simulink model "tracked_vehicle"  (R2026a)
settings: configuration reference "standardSILConfiguraitonParams" (kept outside this file)
undefined symbols (not defined in the file): vehicleParams
settings Model: Creator=jerem  LastModifiedBy=Edison Altamirano
settings ConfigSetRef: SourceName=standardSILConfiguraitonParams  SourceLocation=Base Workspace

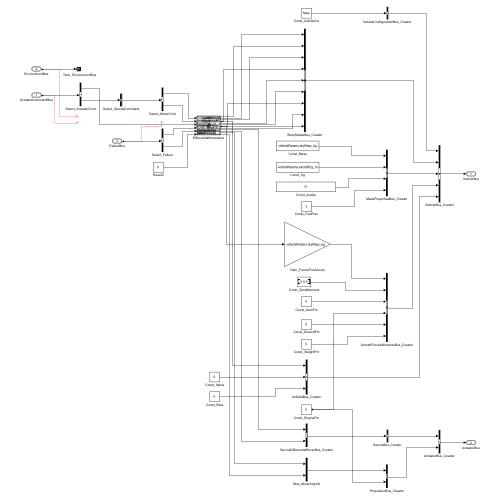
[thumbnail: Simulink's stored preview of the top-level diagram]
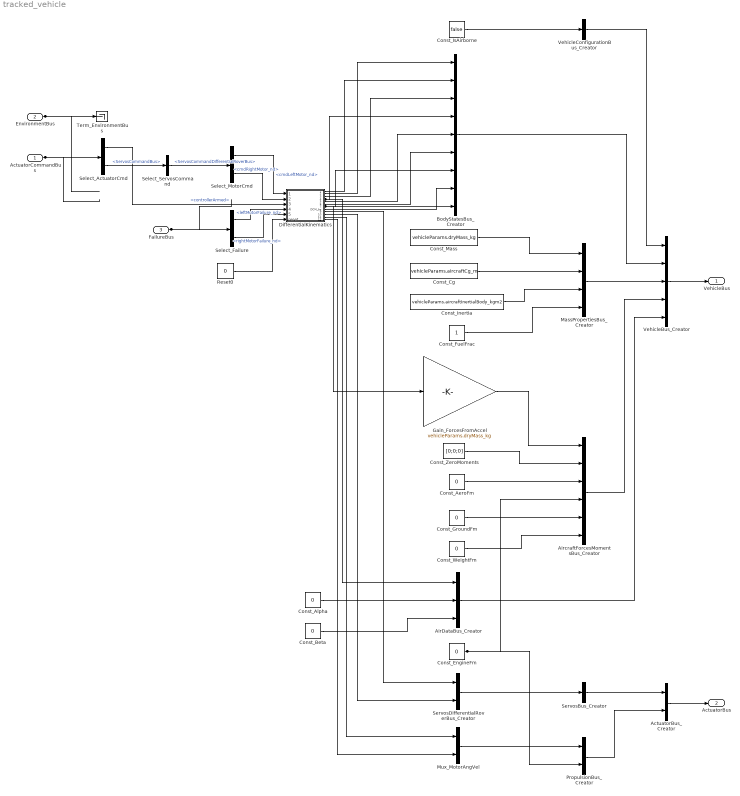
== system tracked_vehicle ==
  ActuatorCommandBus : Inport  OutDataTypeStr=Bus: ActuatorCommandBus
  EnvironmentBus : Inport  Port=2  OutDataTypeStr=Bus: EnvironmentBus
  FailureBus : Inport  Port=3  OutDataTypeStr=Bus: FailureBus
  ActuatorBus_Creator : BusCreator  Inputs=2  OutDataTypeStr=Bus: ActuatorBus
  AirDataBus_Creator : BusCreator  Inputs=3  OutDataTypeStr=Bus: AirDataBus
  AircraftForcesMomentsBus_Creator : BusCreator  Inputs=6  OutDataTypeStr=Bus: AircraftForcesMomentsBus
  BodyStatesBus_Creator : BusCreator  Inputs=9  OutDataTypeStr=Bus: BodyStateBus
  Const_AeroFm : Constant  Value=0  OutDataTypeStr=Bus: ComponentForcesMomentsBus
  Const_Alpha : Constant  Value=0
  Const_Beta : Constant  Value=0
  Const_Cg : Constant  Value=vehicleParams.aircraftCg_m
  Const_EngineFm : Constant  Value=0  OutDataTypeStr=Bus: ComponentForcesMomentsBus
  Const_FuelFrac : Constant
  Const_GroundFm : Constant  Value=0  OutDataTypeStr=Bus: ComponentForcesMomentsBus
  Const_Inertia : Constant  Value=vehicleParams.aircraftInertialBody_kgm2
  Const_IsAirborne : Constant  Value=false  OutDataTypeStr=boolean
  Const_Mass : Constant  Value=vehicleParams.dryMass_kg
  Const_WeightFm : Constant  Value=0  OutDataTypeStr=Bus: ComponentForcesMomentsBus
  Const_ZeroMoments : Constant  Value=[0;0;0]
  DifferentialKinematics : MATLAB Function  TreatAsAtomicUnit=on
  Gain_ForcesFromAccel : Gain  Gain=vehicleParams.dryMass_kg
  MassPropertiesBus_Creator : BusCreator  Inputs=4  OutDataTypeStr=Bus: MassPropertiesBus
  Mux_MotorAngVel : Mux  Inputs=2
  PropulsionBus_Creator : BusCreator  Inputs=2  OutDataTypeStr=Bus: PropulsionBus
  Reset0 : Constant  Value=0
  Select_ActuatorCmd : BusSelector  OutputSignals=controllerArmed,ServosCommandBus
  Select_Failure : BusSelector  OutputSignals=leftMotorFailure_nd,rightMotorFailure_nd
  Select_MotorCmd : BusSelector  OutputSignals=cmdLeftMotor_nd,cmdRightMotor_nd
  Select_ServosCommand : BusSelector  OutputSignals=ServosCommandDifferentialRoverBus
  ServosBus_Creator : BusCreator  Inputs=1  OutDataTypeStr=Bus: ServosBus
  ServosDifferentialRoverBus_Creator : BusCreator  Inputs=2  OutDataTypeStr=Bus: ServosDifferentialRoverBus
  Term_EnvironmentBus : Terminator
  VehicleBus_Creator : BusCreator  Inputs=5  OutDataTypeStr=Bus: VehicleBus
  VehicleConfigurationBus_Creator : BusCreator  Inputs=1  OutDataTypeStr=Bus: VehicleConfigurationBus
  VehicleBus : Outport  OutDataTypeStr=Bus: VehicleBus
  ActuatorBus : Outport  Port=2  OutDataTypeStr=Bus: ActuatorBus
  wires:
  EnvironmentBus/1 -> Term_EnvironmentBus/1
  ActuatorCommandBus/1 -> Select_ActuatorCmd/1
  Const_Mass/1 -> MassPropertiesBus_Creator/1
  Select_ServosCommand/1 -> Select_MotorCmd/1  "<ServosCommandDifferentialRoverBus>"
  Select_ActuatorCmd/1 -> DifferentialKinematics/3(controllerArmed)  "<controllerArmed>"
  Select_ActuatorCmd/2 -> Select_ServosCommand/1  "<ServosCommandBus>"
  Const_Inertia/1 -> MassPropertiesBus_Creator/3
  FailureBus/1 -> Select_Failure/1
  Select_MotorCmd/2 -> DifferentialKinematics/2(cmdRightMotor_nd)  "<cmdRightMotor_nd>"
  PropulsionBus_Creator/1 -> ActuatorBus_Creator/2
  Select_MotorCmd/1 -> DifferentialKinematics/1(cmdLeftMotor_nd)  "<cmdLeftMotor_nd>"
  Select_Failure/1 -> DifferentialKinematics/4(leftMotorFailure_nd)  "<leftMotorFailure_nd>"
  DifferentialKinematics/10(rightWheelSpeed_radps) -> ServosDifferentialRoverBus_Creator/2
  Select_Failure/2 -> DifferentialKinematics/5(rightMotorFailure_nd)  "<rightMotorFailure_nd>"
  Reset0/1 -> DifferentialKinematics/6(reset)
  DifferentialKinematics/1(posNED_m) -> BodyStatesBus_Creator/2
  DifferentialKinematics/2(velNED_mps) -> BodyStatesBus_Creator/1
  DifferentialKinematics/3(eulerAngles_rad) -> BodyStatesBus_Creator/3
  DifferentialKinematics/4(velBody_mps) -> BodyStatesBus_Creator/4, AirDataBus_Creator/1
  AircraftForcesMomentsBus_Creator/1 -> VehicleBus_Creator/4
  Const_EngineFm/1 -> AircraftForcesMomentsBus_Creator/4, PropulsionBus_Creator/2
  DifferentialKinematics/5(angVelBody_radps) -> BodyStatesBus_Creator/5
  DifferentialKinematics/9(leftWheelSpeed_radps) -> ServosDifferentialRoverBus_Creator/1
  DifferentialKinematics/6(angAccelBody_radps2) -> BodyStatesBus_Creator/6
  DifferentialKinematics/7(accelBody_mps2) -> BodyStatesBus_Creator/9, BodyStatesBus_Creator/7, Gain_ForcesFromAccel/1
  DifferentialKinematics/8(DCM_be) -> BodyStatesBus_Creator/8
  VehicleConfigurationBus_Creator/1 -> VehicleBus_Creator/1
  DifferentialKinematics/11(leftMotorAngVel_radps) -> Mux_MotorAngVel/1
  DifferentialKinematics/12(rightMotorAngVel_radps) -> Mux_MotorAngVel/2
  Const_WeightFm/1 -> AircraftForcesMomentsBus_Creator/6
  Const_Alpha/1 -> AirDataBus_Creator/2
  Const_Beta/1 -> AirDataBus_Creator/3
  Const_IsAirborne/1 -> VehicleConfigurationBus_Creator/1
  BodyStatesBus_Creator/1 -> VehicleBus_Creator/2
  Const_Cg/1 -> MassPropertiesBus_Creator/2
  Const_GroundFm/1 -> AircraftForcesMomentsBus_Creator/5
  Const_FuelFrac/1 -> MassPropertiesBus_Creator/4
  ServosBus_Creator/1 -> ActuatorBus_Creator/1
  Gain_ForcesFromAccel/1 -> AircraftForcesMomentsBus_Creator/1
  Const_ZeroMoments/1 -> AircraftForcesMomentsBus_Creator/2
  Const_AeroFm/1 -> AircraftForcesMomentsBus_Creator/3
  AirDataBus_Creator/1 -> VehicleBus_Creator/5
  ServosDifferentialRoverBus_Creator/1 -> ServosBus_Creator/1
  Mux_MotorAngVel/1 -> PropulsionBus_Creator/1
  VehicleBus_Creator/1 -> VehicleBus/1
  MassPropertiesBus_Creator/1 -> VehicleBus_Creator/3
  ActuatorBus_Creator/1 -> ActuatorBus/1

== matlab function tracked_vehicle/DifferentialKinematics ==
  data: cmdLeftMotor_nd input; posNED_m output; cmdRightMotor_nd input; controllerArmed input; leftMotorFailure_nd input; rightMotorFailure_nd input; reset input; velNED_mps output; eulerAngles_rad output; velBody_mps output; angVelBody_radps output; angAccelBody_radps2 output; accelBody_mps2 output; DCM_be output; leftWheelSpeed_radps output; rightWheelSpeed_radps output; leftMotorAngVel_radps output; rightMotorAngVel_radps output
function [posNED_m, velNED_mps, eulerAngles_rad, velBody_mps, angVelBody_radps, angAccelBody_radps2, accelBody_mps2, DCM_be, leftWheelSpeed_radps, rightWheelSpeed_radps, leftMotorAngVel_radps, rightMotorAngVel_radps] = DifferentialKinematics(cmdLeftMotor_nd, cmdRightMotor_nd, controllerArmed, leftMotorFailure_nd, rightMotorFailure_nd, reset)
%#codegen
persistent posN posE yaw leftSpeed rightSpeed
if isempty(posN) || reset
    posN = 0; posE = 0; yaw = 1.9199; leftSpeed = 0; rightSpeed = 0;
end
Ts = 0.004;
trackWidth_m = 1.5;
wheelRadius_m = 0.3;
maxSpeed_mps = 3.0;
tauMotor_s = 0.6;
referenceAltitude_m = 116 * 0.3048;
if leftMotorFailure_nd || ~controllerArmed
    leftCmd_mps = 0;
else
    leftCmd_mps = cmdLeftMotor_nd * maxSpeed_mps;
end
if rightMotorFailure_nd || ~controllerArmed
    rightCmd_mps = 0;
else
    rightCmd_mps = cmdRightMotor_nd * maxSpeed_mps;
end
leftDot = (leftCmd_mps - leftSpeed) / tauMotor_s;
rightDot = (rightCmd_mps - rightSpeed) / tauMotor_s;
v = (leftSpeed + rightSpeed) / 2;
yawRate = (rightSpeed - leftSpeed) / trackWidth_m;
posN = posN + Ts * v * cos(yaw);
posE = posE + Ts * v * sin(yaw);
yaw = yaw + Ts * yawRate;
leftSpeed = leftSpeed + Ts * leftDot;
rightSpeed = rightSpeed + Ts * rightDot;
posNED_m = [posN; posE; -referenceAltitude_m];
velNED_mps = [v*cos(yaw); v*sin(yaw); 0];
eulerAngles_rad = [0; 0; yaw];
velBody_mps = [v; 0; 0];
angVelBody_radps = [0; 0; yawRate];
angAccelBody_radps2 = [0; 0; 0];
vDot = (leftDot + rightDot) / 2;
accelBody_mps2 = [vDot; v*yawRate; 0];
DCM_be = [cos(yaw) sin(yaw) 0; -sin(yaw) cos(yaw) 0; 0 0 1];
leftWheelSpeed_radps = leftSpeed / wheelRadius_m;
rightWheelSpeed_radps = rightSpeed / wheelRadius_m;
leftMotorAngVel_radps = leftWheelSpeed_radps;
rightMotorAngVel_radps = rightWheelSpeed_radps;
